simulink model "cbc_Duffing"  (R2015a)
settings: Solver=ode5  SolverMode=SingleTasking  StartTime=0.0  StopTime=Inf  FixedStep=DeltaT  MaxStep=0.01  RelTol=1e-3
libraries: simulink x2, dsparch4 x1
settings Model: CovSFcnEnable=off  Creator=PD Banneheka  LastModifiedBy=lr14566
settings DataIOCC: SignalLoggingSaveFormat=ModelDataLogs
settings OptimizationCC: BlockReduction=off  OptimizeBlockIOStorage=off  BufferReuse=off  GlobalBufferReuse=off  ExpressionFolding=off  LocalBlockOutputs=off
settings DebuggingCC: ReadBeforeWriteMsg=DisableAll  WriteAfterWriteMsg=DisableAll  WriteAfterReadMsg=DisableAll  UnderspecifiedInitializationDetection=Classic  MergeDetectMultiDrivingBlocksExec=none  SolverPrmCheckMsg=warning  MultiTaskDSMMsg=warning  MultiTaskCondExecSysMsg=none  StateNameClashWarn=warning
settings HardwareCC: ProdBitPerInt=16  ProdBitPerPointer=16  ProdWordSize=16  ProdHWDeviceType=Generic->16-bit Embedded Processor
settings ModelReferenceCC: UpdateModelReferenceTargets=IfOutOfDate  ModelReferenceMinAlgLoopOccurrences=on
settings SFSimCC: SFSimEcho=off

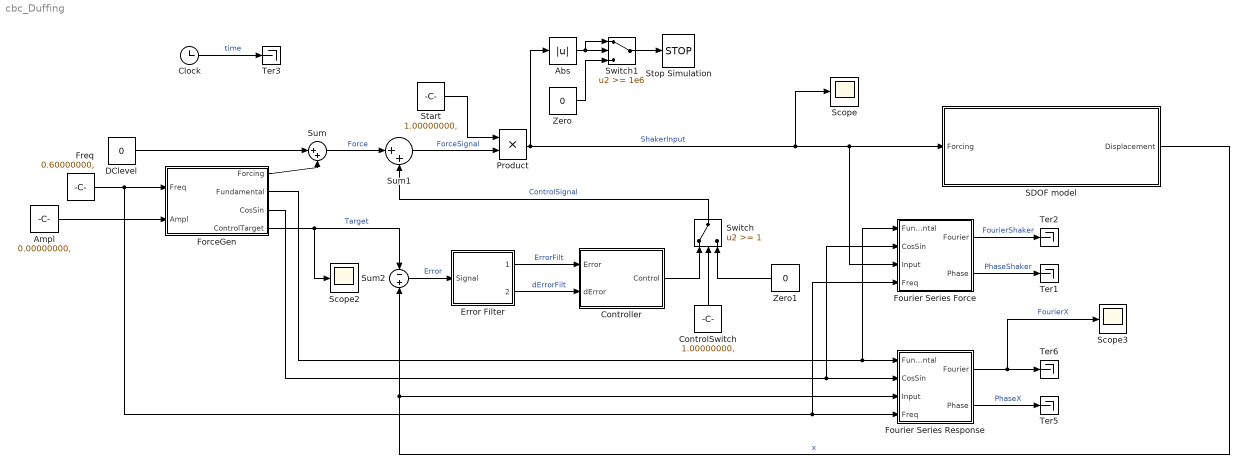
== system cbc_Duffing ==
  Abs : Abs
  Ampl : Constant  Value=0.00000000,
  Clock : Clock
  ControlSwitch : Constant  Value=1.00000000,
  Controller : Subsystem
  DClevel : Constant  Value=0
  Error Filter : Subsystem
  ForceGen : Subsystem
  Fourier Series Force : Subsystem
  Fourier Series Response : Subsystem
  Freq : Constant  Value=0.60000000,  SampleTime=-1
  Product : Product  RndMeth=Zero
  SDOF model : Subsystem
  Scope : Scope
      settings: YMin=-150  YMax=150
  Scope2 : Scope
      settings: YMin=-7.5  YMax=7.5  SaveName=ScopeData2
  Scope3 : Scope
      settings: TimeRange=10  YMin=-0.09  YMax=0.01  SaveName=ScopeData3
  Start : Constant  Value=1.00000000,
  Stop Simulation : Stop
  Sum : Sum  Inputs=|++
  Sum1 : Sum  Inputs=|++
  Sum2 : Sum  Inputs=-|+
  Switch : Switch  Threshold=1
  Switch1 : Switch  Threshold=1e6
  Ter{1..3,5..6} (5 alike) : Terminator
  Zero : Constant  Value=0
  Zero1 : Constant  Value=0
  wires:
  Freq/1 -> ForceGen/1(Freq), Fourier Series Force/4(Freq), Fourier Series Response/4(Freq)
  Ampl/1 -> ForceGen/2(Ampl)
  ForceGen/3(CosSin) -> Fourier Series Force/2(CosSin), Fourier Series Response/2(CosSin)
  ForceGen/2(Fundamental) -> Fourier Series Response/1(Fundamental), Fourier Series Force/1(Fundamental)
  Fourier Series Response/1(Fourier) -> Scope3/1, Ter6/1  "FourierX"
  Fourier Series Response/2(Phase) -> Ter5/1  "PhaseX"
  ForceGen/1(Forcing) -> Sum/2
  SDOF model/1(Displacement) -> Fourier Series Response/3(Input), Sum2/2  "x"
  DClevel/1 -> Sum/1
  Switch1/1 -> Stop Simulation/1
  Abs/1 -> Switch1/2, Switch1/1
  Zero/1 -> Switch1/3
  Start/1 -> Product/1
  Sum/1 -> Sum1/1  "Force"
  Product/1 -> Abs/1, Scope/1, SDOF model/1(Forcing), Fourier Series Force/3(Input)  "ShakerInput"
  Error Filter/1(Filtered) -> Controller/1(Error)  "ErrorFilt"
  Error Filter/2(dFiltered) -> Controller/2(dError)  "dErrorFilt"
  Sum2/1 -> Error Filter/1(Signal)  "Error"
  Controller/1(Control) -> Switch/1
  ControlSwitch/1 -> Switch/2
  Zero1/1 -> Switch/3
  ForceGen/4(ControlTarget) -> Scope2/1, Sum2/1  "Target"
  Sum1/1 -> Product/2  "ForceSignal"
  Switch/1 -> Sum1/2  "ControlSignal"
  Fourier Series Force/1(Fourier) -> Ter2/1  "FourierShaker"
  Fourier Series Force/2(Phase) -> Ter1/1  "PhaseShaker"
  Clock/1 -> Ter3/1  "time"

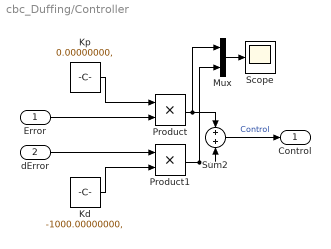
== system cbc_Duffing/Controller ==
  Error : Inport
  dError : Inport  Port=2
  Kd : Constant  Value=-1000.00000000,
  Kp : Constant  Value=0.00000000,
  Mux : Mux  Inputs=2
  Product : Product  RndMeth=Zero
  Product1 : Product  RndMeth=Zero
  Scope : Scope
      settings: TimeRange=10  YMin=-10  YMax=10  SaveName=ScopeData5
  Sum2 : Sum  Inputs=+|+
  Control : Outport
  wires:
  Kp/1 -> Product/1
  Kd/1 -> Product1/2
  Product/1 -> Mux/1, Sum2/1
  Product1/1 -> Sum2/2, Mux/2
  Error/1 -> Product/2
  Sum2/1 -> Control/1  "Control"
  dError/1 -> Product1/1
  Mux/1 -> Scope/1

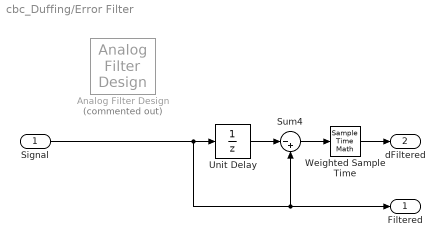
== system cbc_Duffing/Error Filter ==
  Signal : Inport
  Analog Filter Design : dsparch4/Analog Filter Design  Commented=on  method=Butterworth  filttype=Lowpass  N=4  Wlo=2*pi*10  Whi=80  Rp=2  Rs=40
  Sum4 : Sum  Inputs=|-+
  Unit Delay : UnitDelay  SampleTime=-1
  Weighted Sample Time : SampleTimeMath  TsampMathOp=/
  Filtered : Outport
  dFiltered : Outport  Port=2
  wires:
  Unit Delay/1 -> Sum4/1
  Sum4/1 -> Weighted Sample Time/1
  Weighted Sample Time/1 -> dFiltered/1
  Signal/1 -> Unit Delay/1, Filtered/1, Sum4/2

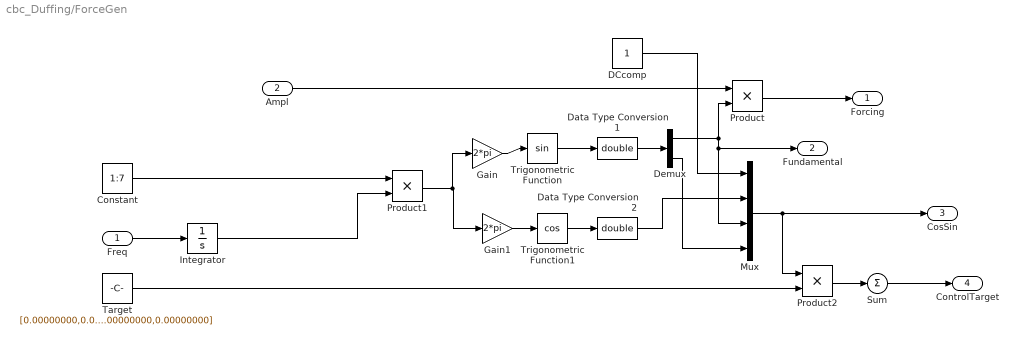
== system cbc_Duffing/ForceGen ==
  Freq : Inport
  Ampl : Inport  Port=2
  Constant : Constant  Value=1:7
  DCcomp : Constant
  Data Type Conversion1 : DataTypeConversion  OutDataTypeStr=double
  Data Type Conversion2 : DataTypeConversion  OutDataTypeStr=double
  Demux : Demux  Outputs=[1,-1]
  Gain : Gain  Gain=2*pi
  Gain1 : Gain  Gain=2*pi
  Integrator : Integrator
  Mux : Mux
  Product : Product
  Product1 : Product
  Product2 : Product  RndMeth=Zero
  Sum : Sum  Inputs=|+|
  Target : Constant  Value=[0.00000000,0.00000000,0.00000000,0.00000000,0.00000000,0.00000000,0.00000000,0.00000000,0.00000000,0.00000000,0.00000000,0.00000000,0.00000000,0.00000000,0.00000000]
  Trigonometric Function : Trigonometry
  Trigonometric Function1 : Trigonometry  Operator=cos
  Forcing : Outport
  Fundamental : Outport  Port=2
  CosSin : Outport  Port=3
  ControlTarget : Outport  Port=4
  wires:
  Freq/1 -> Integrator/1
  Trigonometric Function/1 -> Data Type Conversion1/1
  Data Type Conversion1/1 -> Demux/1
  Ampl/1 -> Product/1
  Product/1 -> Forcing/1
  Constant/1 -> Product1/1
  Product1/1 -> Gain/1, Gain1/1
  Trigonometric Function1/1 -> Data Type Conversion2/1
  Mux/1 -> CosSin/1, Product2/1
  Demux/1 -> Product/2, Fundamental/1, Mux/3
  Integrator/1 -> Product1/2
  Gain/1 -> Trigonometric Function/1
  Gain1/1 -> Trigonometric Function1/1
  Demux/2 -> Mux/4
  Data Type Conversion2/1 -> Mux/2
  DCcomp/1 -> Mux/1
  Product2/1 -> Sum/1
  Sum/1 -> ControlTarget/1
  Target/1 -> Product2/2

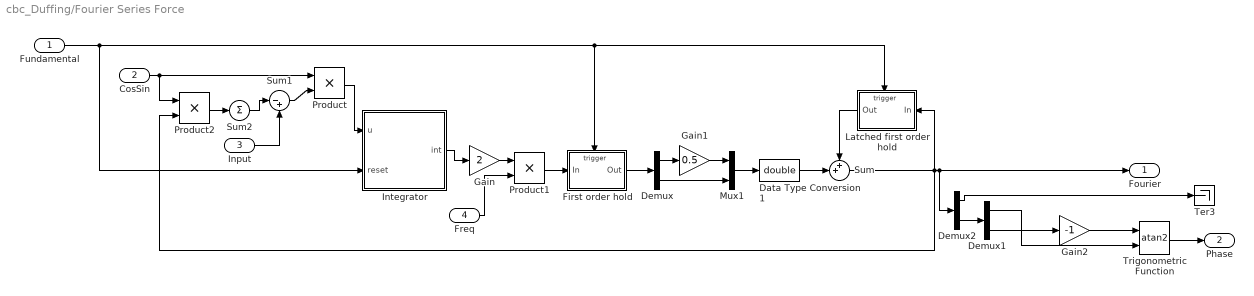
== system cbc_Duffing/Fourier Series Force ==
  Fundamental : Inport
  CosSin : Inport  Port=2
  Input : Inport  Port=3
  Freq : Inport  Port=4
  Data Type Conversion1 : DataTypeConversion  OutDataTypeStr=double
  Demux : Demux  Outputs=[1 -1]
  Demux1 : Demux  Outputs=2
  Demux2 : Demux  Outputs=[1 -1]
  First order hold : Subsystem  TreatAsAtomicUnit=on
  Gain : Gain  Gain=2
  Gain1 : Gain  Gain=0.5
  Gain2 : Gain  Gain=-1
  Integrator : Subsystem
  Latched first order hold : Subsystem  TreatAsAtomicUnit=on
  Mux1 : Mux  Inputs=2
  Product : Product  RndMeth=Zero
  Product1 : Product  RndMeth=Zero
  Product2 : Product  RndMeth=Zero
  Sum : Sum  Inputs=++|
  Sum1 : Sum  Inputs=|-+
  Sum2 : Sum  Inputs=|+|
  Ter3 : Terminator
  Trigonometric Function : Trigonometry  Operator=atan2
  Fourier : Outport
  Phase : Outport  Port=2
  wires:
  Freq/1 -> Product1/2
  Product1/1 -> First order hold/1(In)
  Gain/1 -> Product1/1
  Fundamental/1 -> Integrator/2(reset), First order hold/Trigger, Latched first order hold/Trigger
  Integrator/1(int) -> Gain/1
  Demux/1 -> Gain1/1
  Gain1/1 -> Mux1/1
  Demux/2 -> Mux1/2
  First order hold/1(Out) -> Demux/1
  Mux1/1 -> Data Type Conversion1/1
  Data Type Conversion1/1 -> Sum/2
  Sum/1 -> Product2/2, Latched first order hold/1(In), Fourier/1, Demux2/1
  Latched first order hold/1(Out) -> Sum/1
  Sum1/1 -> Product/2
  Product2/1 -> Sum2/1
  Input/1 -> Sum1/2
  CosSin/1 -> Product/1, Product2/1
  Sum2/1 -> Sum1/1
  Trigonometric Function/1 -> Phase/1
  Product/1 -> Integrator/1(u)
  Demux1/1 -> Trigonometric Function/2
  Demux1/2 -> Gain2/1
  Gain2/1 -> Trigonometric Function/1
  Demux2/2 -> Demux1/1
  Demux2/1 -> Ter3/1

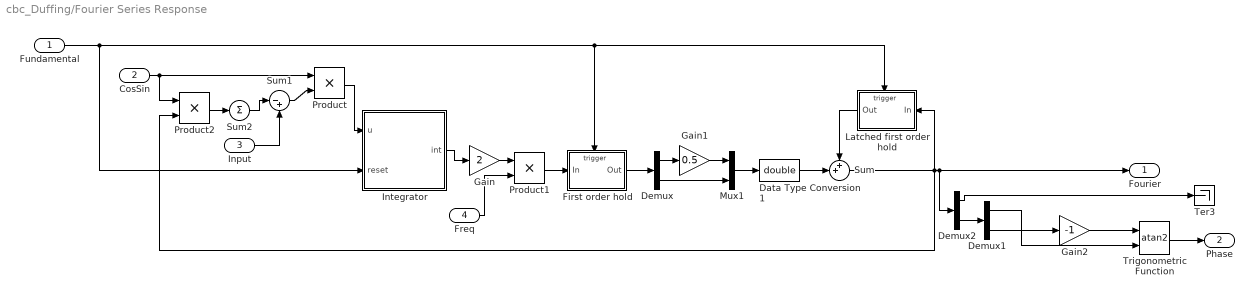
== system cbc_Duffing/Fourier Series Response ==
  Fundamental : Inport
  CosSin : Inport  Port=2
  Input : Inport  Port=3
  Freq : Inport  Port=4
  Data Type Conversion1 : DataTypeConversion  OutDataTypeStr=double
  Demux : Demux  Outputs=[1 -1]
  Demux1 : Demux  Outputs=2
  Demux2 : Demux  Outputs=[1 -1]
  First order hold : Subsystem  TreatAsAtomicUnit=on
  Gain : Gain  Gain=2
  Gain1 : Gain  Gain=0.5
  Gain2 : Gain  Gain=-1
  Integrator : Subsystem
  Latched first order hold : Subsystem  TreatAsAtomicUnit=on
  Mux1 : Mux  Inputs=2
  Product : Product  RndMeth=Zero
  Product1 : Product  RndMeth=Zero
  Product2 : Product  RndMeth=Zero
  Sum : Sum  Tag=Test  Inputs=++|
  Sum1 : Sum  Inputs=|-+
  Sum2 : Sum  Inputs=|+|
  Ter3 : Terminator
  Trigonometric Function : Trigonometry  Operator=atan2
  Fourier : Outport
  Phase : Outport  Port=2
  wires:
  Freq/1 -> Product1/2
  Product1/1 -> First order hold/1(In)
  Gain/1 -> Product1/1
  Fundamental/1 -> Integrator/2(reset), First order hold/Trigger, Latched first order hold/Trigger
  Integrator/1(int) -> Gain/1
  Demux/1 -> Gain1/1
  Gain1/1 -> Mux1/1
  Demux/2 -> Mux1/2
  First order hold/1(Out) -> Demux/1
  Mux1/1 -> Data Type Conversion1/1
  Data Type Conversion1/1 -> Sum/2
  Sum/1 -> Product2/2, Latched first order hold/1(In), Fourier/1, Demux2/1
  Latched first order hold/1(Out) -> Sum/1
  Sum1/1 -> Product/2
  Product2/1 -> Sum2/1
  Input/1 -> Sum1/2
  CosSin/1 -> Product/1, Product2/1
  Sum2/1 -> Sum1/1
  Trigonometric Function/1 -> Phase/1
  Product/1 -> Integrator/1(u)
  Demux1/1 -> Trigonometric Function/2
  Demux1/2 -> Gain2/1
  Gain2/1 -> Trigonometric Function/1
  Demux2/2 -> Demux1/1
  Demux2/1 -> Ter3/1

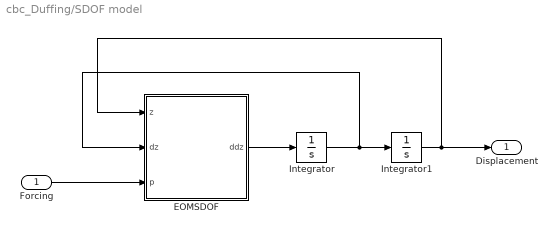
== system cbc_Duffing/SDOF model ==
  Forcing : Inport
  EOMSDOF : Subsystem
  Integrator : Integrator
  Integrator1 : Integrator  InitialCondition=1
  Displacement : Outport
  wires:
  EOMSDOF/1(ddz) -> Integrator/1
  Integrator/1 -> EOMSDOF/2(dz), Integrator1/1
  Forcing/1 -> EOMSDOF/3(p)
  Integrator1/1 -> Displacement/1, EOMSDOF/1(z)

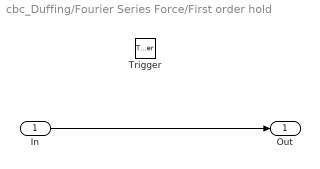
== system cbc_Duffing/Fourier Series Force/First order hold ==
  In : Inport  LatchByDelayingOutsideSignal=on
  Trigger : TriggerPort
  Out : Outport
  wires:
  In/1 -> Out/1

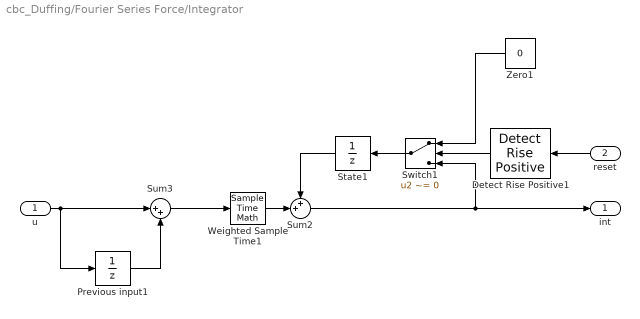
== system cbc_Duffing/Fourier Series Force/Integrator ==
  u : Inport
  reset : Inport  Port=2
  Detect Rise Positive1 : simulink/Logic and Bit Operations/Detect Rise Positive  vinit=0  InputProcessing=Inherited  OutDataTypeStr=uint8
  Previous input1 : UnitDelay  SampleTime=-1
  State1 : UnitDelay  SampleTime=-1
  Sum2 : Sum  Inputs=++|
  Sum3 : Sum  Inputs=|++
  Switch1 : Switch  Criteria=u2 ~= 0
  Weighted Sample Time1 : SampleTimeMath  TsampMathOp=*  weightValue=0.5
  Zero1 : Constant  Value=0
  int : Outport
  wires:
  Detect Rise Positive1/1 -> Switch1/2
  Zero1/1 -> Switch1/1
  Switch1/1 -> State1/1
  reset/1 -> Detect Rise Positive1/1
  Previous input1/1 -> Sum3/2
  u/1 -> Previous input1/1, Sum3/1
  Sum3/1 -> Weighted Sample Time1/1
  Weighted Sample Time1/1 -> Sum2/2
  Sum2/1 -> int/1, Switch1/3
  State1/1 -> Sum2/1

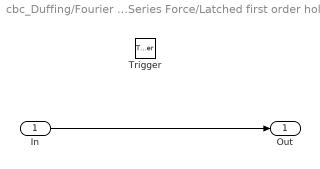
== system cbc_Duffing/Fourier Series Force/Latched first order hold ==
  In : Inport  LatchByDelayingOutsideSignal=on
  Trigger : TriggerPort
  Out : Outport
  wires:
  In/1 -> Out/1

== system cbc_Duffing/Fourier Series Response/First order hold ==
  In : Inport  LatchByDelayingOutsideSignal=on
  Trigger : TriggerPort
  Out : Outport
  wires:
  In/1 -> Out/1

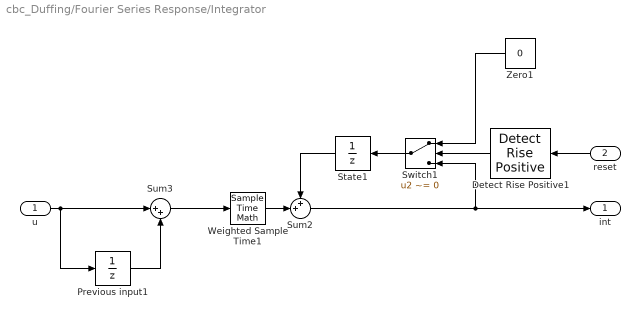
== system cbc_Duffing/Fourier Series Response/Integrator ==
  u : Inport
  reset : Inport  Port=2
  Detect Rise Positive1 : simulink/Logic and Bit Operations/Detect Rise Positive  vinit=0  InputProcessing=Inherited  OutDataTypeStr=uint8
  Previous input1 : UnitDelay  SampleTime=-1
  State1 : UnitDelay  SampleTime=-1
  Sum2 : Sum  Inputs=++|
  Sum3 : Sum  Inputs=|++
  Switch1 : Switch  Criteria=u2 ~= 0
  Weighted Sample Time1 : SampleTimeMath  TsampMathOp=*  weightValue=0.5
  Zero1 : Constant  Value=0
  int : Outport
  wires:
  Detect Rise Positive1/1 -> Switch1/2
  Zero1/1 -> Switch1/1
  Switch1/1 -> State1/1
  reset/1 -> Detect Rise Positive1/1
  Previous input1/1 -> Sum3/2
  u/1 -> Previous input1/1, Sum3/1
  Sum3/1 -> Weighted Sample Time1/1
  Weighted Sample Time1/1 -> Sum2/2
  Sum2/1 -> int/1, Switch1/3
  State1/1 -> Sum2/1

== system cbc_Duffing/Fourier Series Response/Latched first order hold ==
  In : Inport  LatchByDelayingOutsideSignal=on
  Trigger : TriggerPort
  Out : Outport
  wires:
  In/1 -> Out/1

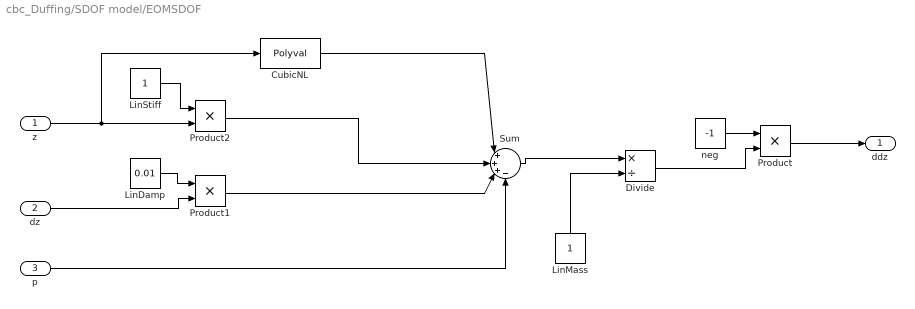
== system cbc_Duffing/SDOF model/EOMSDOF ==
  z : Inport
  dz : Inport  Port=2
  p : Inport  Port=3
  CubicNL : Polyval  Coefs=[0.5,0,0,0]
  Divide : Product  Inputs=*/
  LinDamp : Constant  Value=0.01
  LinMass : Constant
  LinStiff : Constant
  Product : Product
  Product1 : Product
  Product2 : Product
  Sum : Sum  Inputs=|+++-
  neg : Constant  Value=-1
  ddz : Outport
  wires:
  Product/1 -> ddz/1
  neg/1 -> Product/1
  LinMass/1 -> Divide/2
  Sum/1 -> Divide/1
  Divide/1 -> Product/2
  z/1 -> CubicNL/1, Product2/2
  LinStiff/1 -> Product2/1
  dz/1 -> Product1/2
  LinDamp/1 -> Product1/1
  Product2/1 -> Sum/2
  Product1/1 -> Sum/3
  p/1 -> Sum/4
  CubicNL/1 -> Sum/1
